simulink model "LQR_control"  (R2020b)
settings: Solver=ode4  StartTime=0.0  StopTime=SIM_TIME  FixedStep=STEP_SIZE  RelTol=1e-3
undefined symbols (not defined in the file): A_0, A_step, c1, c2, f1, f2, f3, f4, f5, f6, g, Ki, Kx, m, t_step, Ts, uss, xss, yss
settings Model: Creator=Roberto  LastModifiedBy=maxfi
settings DataIOCC: ReturnWorkspaceOutputs=off
settings DebuggingCC: ArithmeticOperatorsInVariantConditions=warning
settings SFSimCC: SimUseLocalCustomCode=off  CustomCodeUndefinedFunction=UseInterfaceOnly
settings RTWCC: RTWUseLocalCustomCode=off
settings CodeAppCC: StateflowObjectComments=on

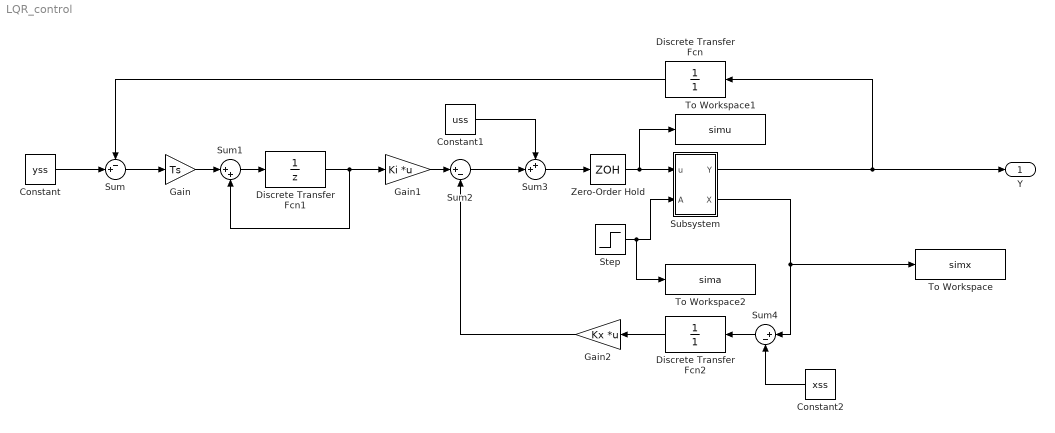
== system LQR_control ==
  Constant : Constant  Value=yss
  Constant1 : Constant  Value=uss
  Constant2 : Constant  Value=xss
  Discrete Transfer Fcn : DiscreteTransferFcn  Denominator=[1]  SampleTime=Ts
  Discrete Transfer Fcn1 : DiscreteTransferFcn  Denominator=[1 0]  SampleTime=Ts
  Discrete Transfer Fcn2 : DiscreteTransferFcn  Denominator=[1]  SampleTime=Ts
  Gain : Gain  Gain=Ts
  Gain1 : Gain  Gain=Ki  Multiplication=Matrix(K*u)
  Gain2 : Gain  Gain=Kx  Multiplication=Matrix(K*u)
  Step : Step  Time=t_step  Before=A_0  After=A_step  SampleTime=0
  Subsystem : Subsystem
  Sum : Sum  Inputs=-+|
  Sum1 : Sum  Inputs=|++
  Sum2 : Sum  Inputs=|+-
  Sum3 : Sum  Inputs=++|
  Sum4 : Sum  Inputs=|+-
  To Workspace : ToWorkspace  VariableName=simx  SaveFormat=Structure With Time  SampleTime=-1
  To Workspace1 : ToWorkspace  VariableName=simu  SaveFormat=Structure With Time  SampleTime=-1
  To Workspace2 : ToWorkspace  VariableName=sima  SaveFormat=Structure With Time  SampleTime=-1
  Zero-Order Hold : ZeroOrderHold  SampleTime=Ts
  Y : Outport  VectorParamsAs1DForOutWhenUnconnected=off
  wires:
  Step/1 -> To Workspace2/1, Subsystem/2(A)
  Subsystem/1(Y) -> Discrete Transfer Fcn/1, Y/1
  Constant/1 -> Sum/2
  Discrete Transfer Fcn/1 -> Sum/1
  Sum/1 -> Gain/1
  Gain/1 -> Sum1/1
  Sum1/1 -> Discrete Transfer Fcn1/1
  Discrete Transfer Fcn1/1 -> Gain1/1, Sum1/2
  Gain1/1 -> Sum2/1
  Sum2/1 -> Sum3/2
  Constant1/1 -> Sum3/1
  Sum3/1 -> Zero-Order Hold/1
  Zero-Order Hold/1 -> To Workspace1/1, Subsystem/1(u)
  Subsystem/2(X) -> To Workspace/1, Sum4/1
  Constant2/1 -> Sum4/2
  Sum4/1 -> Discrete Transfer Fcn2/1
  Discrete Transfer Fcn2/1 -> Gain2/1
  Gain2/1 -> Sum2/2

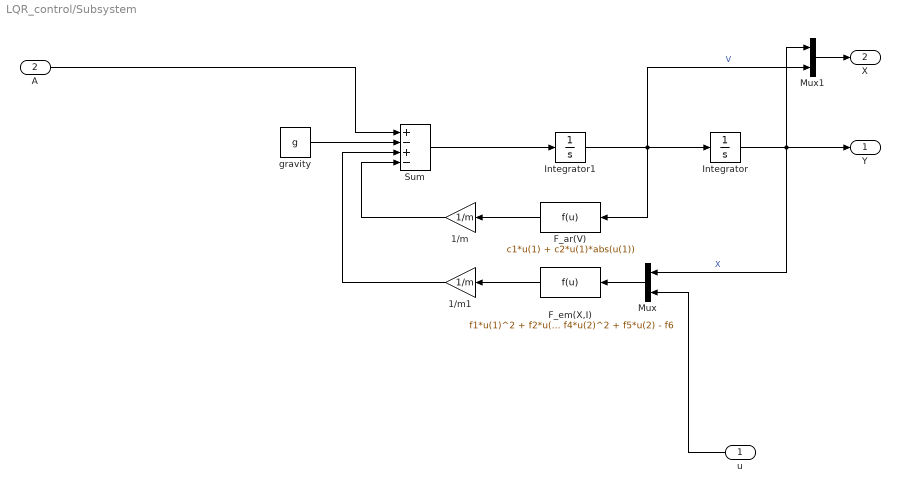
== system LQR_control/Subsystem ==
  u : Inport
  A : Inport  Port=2
  1/m : Gain  Gain=1/m
  1/m1 : Gain  Gain=1/m
  F_ar(V) : Fcn  Expr=c1*u(1) + c2*u(1)*abs(u(1))
  F_em(X,I) : Fcn  Expr=f1*u(1)^2 + f2*u(1)*u(2) - f3*u(1) + f4*u(2)^2 + f5*u(2) - f6
  Integrator : Integrator  Priority=1  InitialCondition=xss(1)
  Integrator1 : Integrator  Priority=2  InitialCondition=xss(2)
  Mux : Mux  Inputs=2
  Mux1 : Mux  Inputs=2
  Sum : Sum  Inputs=+-+-
  gravity : Constant  Value=g
  Y : Outport
  X : Outport  Port=2
  wires:
  Integrator/1 -> Mux1/1, Y/1, Mux/1  "X"
  F_em(X,I)/1 -> 1/m1/1
  Mux/1 -> F_em(X,I)/1
  1/m1/1 -> Sum/3
  Integrator1/1 -> Mux1/2, Integrator/1, F_ar(V)/1  "V"
  gravity/1 -> Sum/2
  Sum/1 -> Integrator1/1
  1/m/1 -> Sum/4
  F_ar(V)/1 -> 1/m/1
  A/1 -> Sum/1
  u/1 -> Mux/2
  Mux1/1 -> X/1
